simulink library "PTOSim_Lib"  (R2014b)
settings: Solver=ode45  StartTime=0.0  StopTime=10.0  RelTol=1e-3
undefined symbols (not defined in the file): alpha, Amax, Amin, Ap, Beta_e, bf, bg, Cd, D, driveEff, J, k1, k2, omegaBase, omegaInit, pAeq, pAi, pAupper_limit, pBeq, pBi, pBupper_limit, pCprecharge, pDprecharge, pMax, pMin, rho, simu, TgenBase, tot, VC0, VCeq, VD0, VDeq, Vo
libraries: PTOSim_Lib x7, WECSim_Lib x2
settings Model: Creator=sor  LastModifiedBy=sor

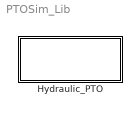
== system PTOSim_Lib ==
  Hydraulic_PTO : Subsystem  RequirementInfo={} %GIDa_f12a42eb_b9cb_4818_b573_b7dee4183a3b

== system PTOSim_Lib/Hydraulic_PTO ==
  Accumulator : Subsystem  Variant=on  mask{pto=0}
      mask prompts: pto "PTO Name"
  Generator : Subsystem  RequirementInfo="{}  %GIDa_30368e1c_dc2a_4605_bb50_ff3a423f2df5"  mask{pto=0}
      mask prompts: pto "PTO Name"
  "Motor " : Subsystem  mask{pto=0}
      mask prompts: pto "PTO Name"
  PTOSIM : Subsystem  RequirementInfo="{}  %GIDa_b8f519ee_1776_4469_9852_74bfa511eadd"  mask{Parameter1=0}
      mask prompts: Parameter1 "pto"
  "Piston " : Subsystem  mask{pto=0}
      mask prompts: pto "PTO Name"
  Piston 1 : PTOSim_Lib/Hydraulic_PTO/Piston    pto=0
  Rectifiying Check Valve : Subsystem  RequirementInfo="{}  %GIDa_a75844df_5079_4f47_95bd_8083cdfec0d7"  mask{pto=0}
      mask prompts: pto "PTO Name"

== system PTOSim_Lib/Hydraulic_PTO/Accumulator ==
  note: 1) Only subsystems can be added as variant choices at this level
      | 2) Blocks cannot be connected at this level as connectivity is
      | automatically determined at simulation, based on the active variant
  Vdot : Inport
  Vdotm : Inport  Port=2
  High Pressure Accumulator : Subsystem  VariantControl=Variant
  Low Pressure Accumulator : Subsystem  VariantControl=Variant1
  Pressure : Outport

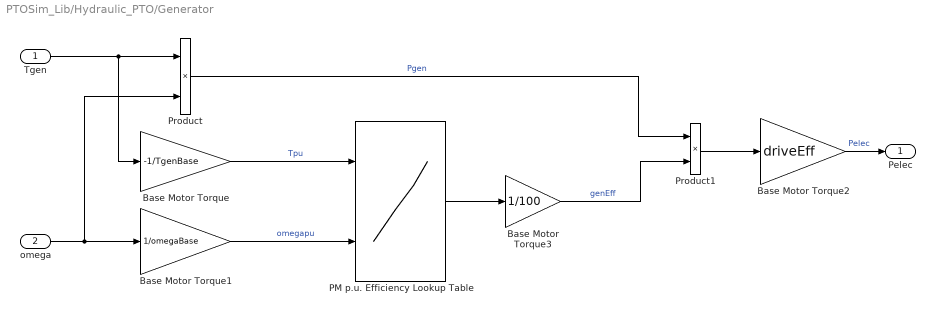
== system PTOSim_Lib/Hydraulic_PTO/Generator ==
  Tgen : Inport
  omega : Inport  Port=2
  Base Motor Torque : Gain  Gain=-1/TgenBase
  Base Motor Torque1 : Gain  Gain=1/omegaBase
  Base Motor Torque2 : Gain  Gain=driveEff
  Base Motor Torque3 : Gain  Gain=1/100
  PM p.u. Efficiency Lookup Table : Lookup_n-D  BreakpointsForDimension1=tot.Tpu(:,1)  BreakpointsForDimension2=tot.omegapu(1,:)  Table=tot.eff  InterpMethod=Flat  InputSameDT=on
  Product : Product  RndMeth=Zero
  Product1 : Product  RndMeth=Zero
  Pelec : Outport
  wires:
  Base Motor Torque2/1 -> Pelec/1  "Pelec"
  Product1/1 -> Base Motor Torque2/1
  Product/1 -> Product1/1  "Pgen"
  Base Motor Torque3/1 -> Product1/2  "genEff"
  PM p.u. Efficiency Lookup Table/1 -> Base Motor Torque3/1
  omega/1 -> Product/2, Base Motor Torque1/1
  Base Motor Torque1/1 -> PM p.u. Efficiency Lookup Table/2  "omegapu"
  Tgen/1 -> Base Motor Torque/1, Product/1
  Base Motor Torque/1 -> PM p.u. Efficiency Lookup Table/1  "Tpu"

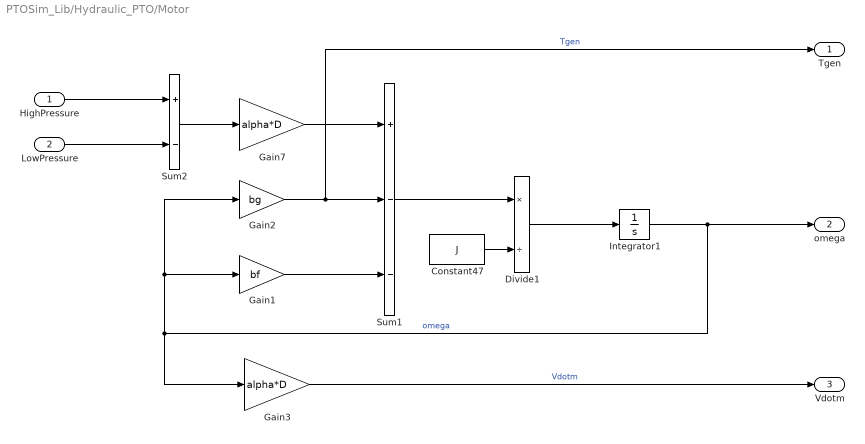
== system PTOSim_Lib/Hydraulic_PTO/Motor  ==
  HighPressure : Inport
  LowPressure : Inport  Port=2
  Constant47 : Constant  Value=J
  Divide1 : Product  Inputs=*/
  Gain1 : Gain  Gain=bf
  Gain2 : Gain  Gain=bg
  Gain3 : Gain  Gain=alpha*D
  Gain7 : Gain  Gain=alpha*D
  Integrator1 : Integrator  InitialCondition=omegaInit
  Sum1 : Sum  Inputs=+--
  Sum2 : Sum  Inputs=+-
  Tgen : Outport
  omega : Outport  Port=2
  Vdotm : Outport  Port=3
  wires:
  Gain7/1 -> Sum1/1
  Gain2/1 -> Tgen/1, Sum1/2  "Tgen"
  Gain1/1 -> Sum1/3
  Sum1/1 -> Divide1/1
  Constant47/1 -> Divide1/2
  Divide1/1 -> Integrator1/1
  Integrator1/1 -> omega/1, Gain3/1, Gain1/1, Gain2/1  "omega"
  Gain3/1 -> Vdotm/1  "Vdotm"
  HighPressure/1 -> Sum2/1
  LowPressure/1 -> Sum2/2
  Sum2/1 -> Gain7/1

== system PTOSim_Lib/Hydraulic_PTO/PTOSIM ==
  zRel : Inport
  zDotRel : Inport  Port=2
  Accumulator : PTOSim_Lib/Hydraulic_PTO/Accumulator  OverrideUsingVariant=Variant  pto=0
  Accumulator1 : PTOSim_Lib/Hydraulic_PTO/Accumulator  OverrideUsingVariant=Variant1  pto=0
  Generator : PTOSim_Lib/Hydraulic_PTO/Generator  pto=0
  "Motor " : PTOSim_Lib/Hydraulic_PTO/Motor   pto=0
  "Piston " : PTOSim_Lib/Hydraulic_PTO/Piston    pto=0
  Rectifiying Check Valve : PTOSim_Lib/Hydraulic_PTO/Rectifiying  Check Valve  pto=0
  Terminator : Terminator
  Fpto : Outport
  wires:
  zRel/1 -> "Piston "/1  "zRel"
  zDotRel/1 -> "Piston "/2  "zDotRel"
  "Piston "/2 -> Rectifiying Check Valve/1  "TopPistonPressure"
  "Piston "/3 -> Rectifiying Check Valve/2  "BottomPistonPressure"
  "Motor "/1 -> Generator/1
  "Motor "/2 -> Generator/2
  "Motor "/3 -> Accumulator/2, Accumulator1/2
  Accumulator/1 -> Rectifiying Check Valve/3, "Motor "/1  "HighPressure"
  Accumulator1/1 -> "Motor "/2, Rectifiying Check Valve/4  "LowPressure"
  Rectifiying Check Valve/1 -> "Piston "/3, Accumulator1/1, Accumulator/1
  Generator/1 -> Terminator/1
  "Piston "/1 -> Fpto/1

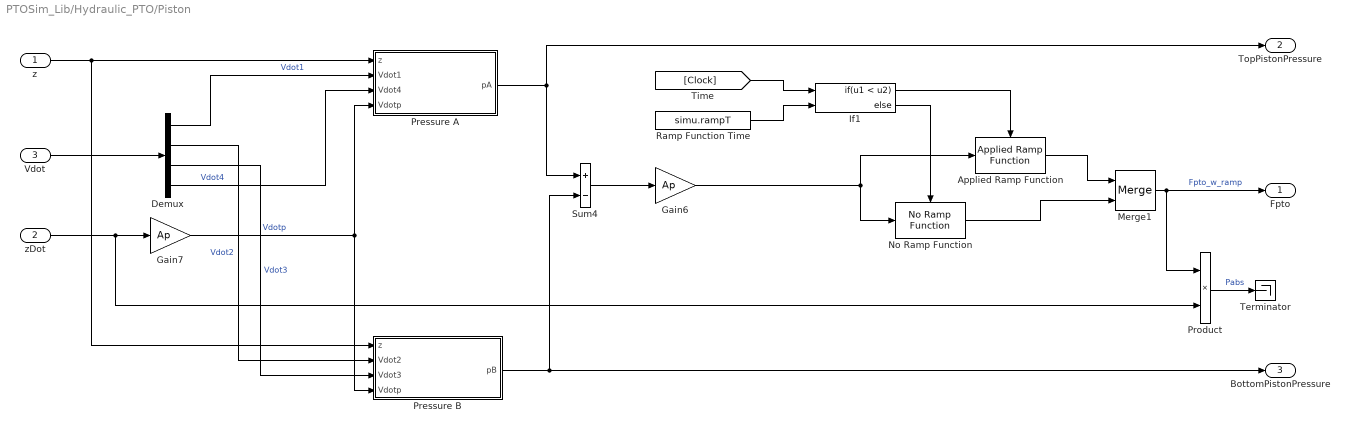
== system PTOSim_Lib/Hydraulic_PTO/Piston  ==
  z : Inport
  zDot : Inport  Port=2
  Vdot : Inport  Port=3
  Applied Ramp Function : WECSim_Lib/Body Elements/Rigid Body/Wave Diffraction and Excitation Force Calculation/Applied Ramp Function
  Demux : Demux
  Gain6 : Gain  Gain=Ap
  Gain7 : Gain  Gain=Ap
  If1 : If  NumInputs=2  IfExpression=u1 < u2
  Merge1 : Merge
  No Ramp Function : WECSim_Lib/Body Elements/Rigid Body/Wave Diffraction and Excitation Force Calculation/No Ramp Function
  Pressure A : Subsystem
  Pressure B : Subsystem  RequirementInfo="{}  %GIDa_18ee15fe_6148_4b69_b054_be19d4b47378"
  Product : Product
  Ramp Function Time : Constant  Value=simu.rampT
  Sum4 : Sum  Inputs=+-
  Terminator : Terminator
  Fpto : Outport
  TopPistonPressure : Outport  Port=2
  BottomPistonPressure : Outport  Port=3
  wires:
  Pressure A/1(pA) -> TopPistonPressure/1, Sum4/1
  Pressure B/1(pB) -> Sum4/2, BottomPistonPressure/1
  Gain7/1 -> Pressure B/4(Vdotp), Pressure A/4(Vdotp)  "Vdotp"
  Gain6/1 -> No Ramp Function/1, Applied Ramp Function/1
  Product/1 -> Terminator/1  "Pabs"
  Vdot/1 -> Demux/1
  z/1 -> Pressure B/1(z), Pressure A/1(z)
  Demux/1 -> Pressure A/2(Vdot1)  "Vdot1"
  Demux/2 -> Pressure B/2(Vdot2)  "Vdot2"
  Demux/3 -> Pressure B/3(Vdot3)  "Vdot3"
  Demux/4 -> Pressure A/3(Vdot4)  "Vdot4"
  Sum4/1 -> Gain6/1
  If1/1 -> Applied Ramp Function/Action
  If1/2 -> No Ramp Function/Action
  Applied Ramp Function/1 -> Merge1/1
  No Ramp Function/1 -> Merge1/2
  Merge1/1 -> Product/1, Fpto/1  "Fpto_w_ramp"
  [Clock] -> If1/1
  Ramp Function Time/1 -> If1/2
  zDot/1 -> Product/2, Gain7/1

== system PTOSim_Lib/Hydraulic_PTO/Rectifiying Check Valve ==
  TopPistonPressure : Inport
  BottomPistonPressure : Inport  Port=2
  HighPressure : Inport  Port=3
  LowPressure : Inport  Port=4
  Bus Creator : BusCreator
  Subsystem : Subsystem  RequirementInfo="{}  %GIDa_43e7490a_26e5_4c96_a755_05599e7ab58d"
  Subsystem1 : Subsystem
  Subsystem2 : Subsystem
  Subsystem3 : Subsystem  RequirementInfo="{}  %GIDa_1d14c02d_1c58_4958_a821_20fe782ea22d"
  Vdot : Outport
  wires:
  TopPistonPressure/1 -> Subsystem3/2(pA), Subsystem/1(pA)
  BottomPistonPressure/1 -> Subsystem2/2(pB), Subsystem1/1(pB)
  HighPressure/1 -> Subsystem1/2(pC), Subsystem/2(pC)
  LowPressure/1 -> Subsystem3/1(pD), Subsystem2/1(pD)
  Subsystem3/1(Vdot4) -> Bus Creator/4  "Vdot4"
  Subsystem2/1(Vdot3) -> Bus Creator/3  "Vdot3"
  Subsystem1/1(Vdot2) -> Bus Creator/2  "Vdot2"
  Subsystem/1(Vdot1) -> Bus Creator/1  "Vdot1"
  Bus Creator/1 -> Vdot/1

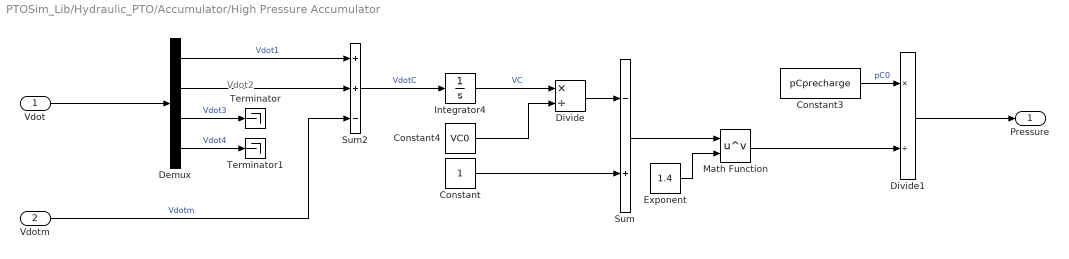
== system PTOSim_Lib/Hydraulic_PTO/Accumulator/High Pressure Accumulator ==
  note: Vdot2
  Vdot : Inport
  Vdotm : Inport  Port=2
  Constant : Constant
  Constant3 : Constant  Value=pCprecharge
  Constant4 : Constant  Value=VC0
  Demux : Demux
  Divide : Product  Inputs=*/
  Divide1 : Product  Inputs=*/
  Exponent : Constant  Value=1.4
  Integrator4 : Integrator  InitialCondition=VCeq
  Math Function : Math  Operator=pow  SaturateOnIntegerOverflow=on
  Sum : Sum  Inputs=-+
  Sum2 : Sum  Inputs=++-
  Terminator : Terminator
  Terminator1 : Terminator
  Pressure : Outport
  wires:
  Sum2/1 -> Integrator4/1  "VdotC"
  Integrator4/1 -> Divide/1  "VC"
  Constant4/1 -> Divide/2
  Constant/1 -> Sum/2
  Divide/1 -> Sum/1
  Exponent/1 -> Math Function/2
  Sum/1 -> Math Function/1
  Math Function/1 -> Divide1/2
  Constant3/1 -> Divide1/1  "pC0"
  Divide1/1 -> Pressure/1
  Vdot/1 -> Demux/1
  Demux/3 -> Terminator/1  "Vdot3"
  Demux/4 -> Terminator1/1  "Vdot4"
  Demux/1 -> Sum2/1  "Vdot1"
  Demux/2 -> Sum2/2
  Vdotm/1 -> Sum2/3  "Vdotm"

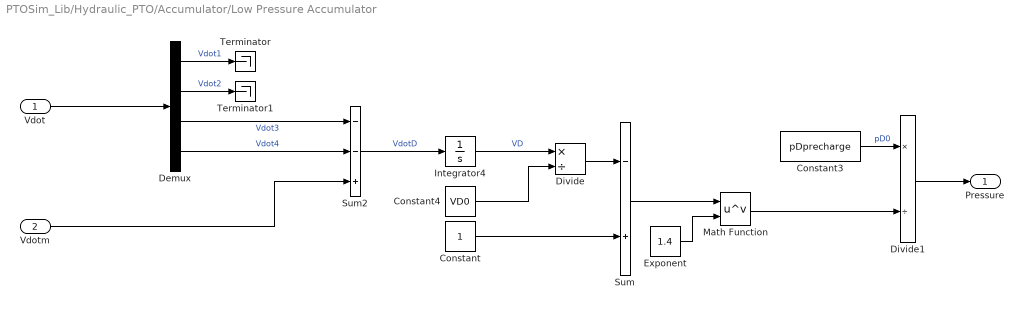
== system PTOSim_Lib/Hydraulic_PTO/Accumulator/Low Pressure Accumulator ==
  Vdot : Inport
  Vdotm : Inport  Port=2
  Constant : Constant
  Constant3 : Constant  Value=pDprecharge
  Constant4 : Constant  Value=VD0
  Demux : Demux
  Divide : Product  Inputs=*/
  Divide1 : Product  Inputs=*/
  Exponent : Constant  Value=1.4
  Integrator4 : Integrator  InitialCondition=VDeq
  Math Function : Math  Operator=pow  SaturateOnIntegerOverflow=on
  Sum : Sum  Inputs=-+
  Sum2 : Sum  Inputs=--+
  Terminator : Terminator
  Terminator1 : Terminator
  Pressure : Outport
  wires:
  Sum2/1 -> Integrator4/1  "VdotD"
  Integrator4/1 -> Divide/1  "VD"
  Constant4/1 -> Divide/2
  Constant/1 -> Sum/2
  Divide/1 -> Sum/1
  Exponent/1 -> Math Function/2
  Sum/1 -> Math Function/1
  Math Function/1 -> Divide1/2
  Constant3/1 -> Divide1/1  "pD0"
  Divide1/1 -> Pressure/1
  Vdot/1 -> Demux/1
  Demux/3 -> Sum2/1  "Vdot3"
  Demux/4 -> Sum2/2  "Vdot4"
  Vdotm/1 -> Sum2/3
  Demux/1 -> Terminator/1  "Vdot1"
  Demux/2 -> Terminator1/1  "Vdot2"

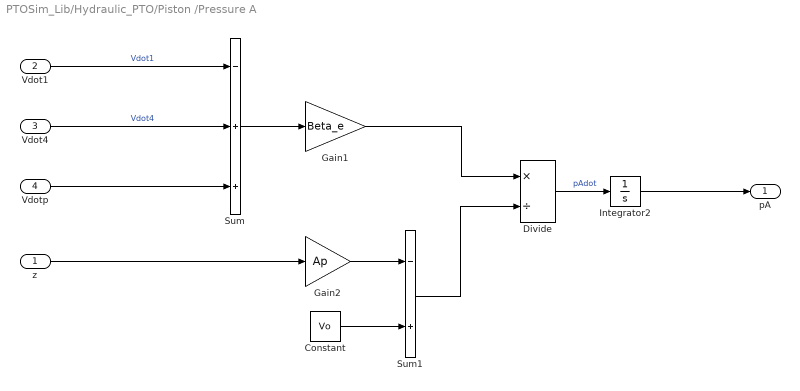
== system PTOSim_Lib/Hydraulic_PTO/Piston /Pressure A ==
  z : Inport
  Vdot1 : Inport  Port=2
  Vdot4 : Inport  Port=3
  Vdotp : Inport  Port=4
  Constant : Constant  Value=Vo
  Divide : Product  Inputs=*/
  Gain1 : Gain  Gain=Beta_e
  Gain2 : Gain  Gain=Ap
  Integrator2 : Integrator  InitialCondition=pAi  UpperSaturationLimit=pAupper_limit  LowerSaturationLimit=pAeq
  Sum : Sum  Inputs=-++
  Sum1 : Sum  Inputs=-+
  pA : Outport
  wires:
  Sum/1 -> Gain1/1
  z/1 -> Gain2/1
  Gain2/1 -> Sum1/1
  Constant/1 -> Sum1/2
  Gain1/1 -> Divide/1
  Sum1/1 -> Divide/2
  Vdot1/1 -> Sum/1  "Vdot1"
  Divide/1 -> Integrator2/1  "pAdot"
  Vdot4/1 -> Sum/2  "Vdot4"
  Integrator2/1 -> pA/1
  Vdotp/1 -> Sum/3

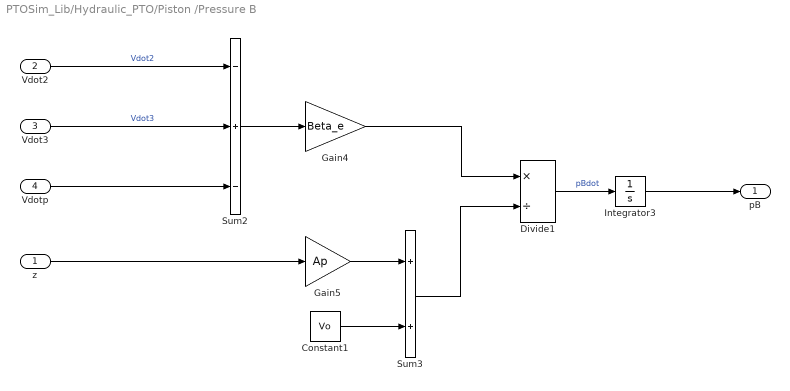
== system PTOSim_Lib/Hydraulic_PTO/Piston /Pressure B ==
  z : Inport
  Vdot2 : Inport  Port=2
  Vdot3 : Inport  Port=3
  Vdotp : Inport  Port=4
  Constant1 : Constant  Value=Vo
  Divide1 : Product  Inputs=*/
  Gain4 : Gain  Gain=Beta_e
  Gain5 : Gain  Gain=Ap
  Integrator3 : Integrator  InitialCondition=pBi  UpperSaturationLimit=pBupper_limit  LowerSaturationLimit=pBeq
  Sum2 : Sum  Inputs=-+-
  Sum3 : Sum
  pB : Outport
  wires:
  Sum2/1 -> Gain4/1
  z/1 -> Gain5/1
  Gain5/1 -> Sum3/1
  Constant1/1 -> Sum3/2
  Gain4/1 -> Divide1/1
  Sum3/1 -> Divide1/2
  Divide1/1 -> Integrator3/1  "pBdot"
  Vdot2/1 -> Sum2/1  "Vdot2"
  Vdot3/1 -> Sum2/2  "Vdot3"
  Integrator3/1 -> pB/1
  Vdotp/1 -> Sum2/3

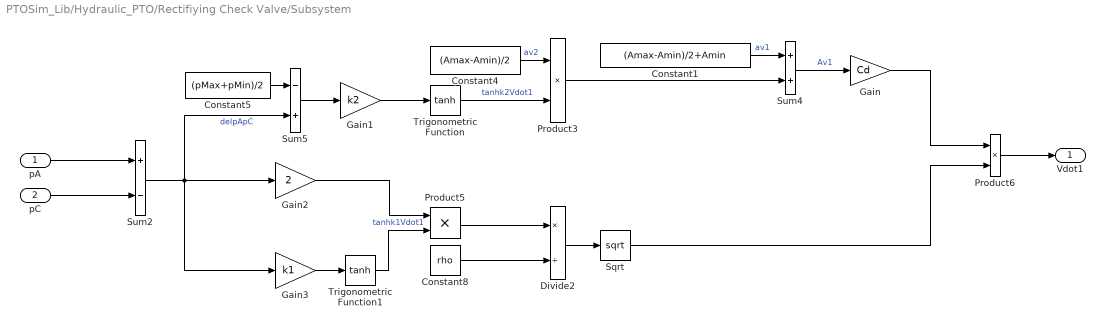
== system PTOSim_Lib/Hydraulic_PTO/Rectifiying Check Valve/Subsystem ==
  pA : Inport
  pC : Inport  Port=2
  Constant1 : Constant  Value=(Amax-Amin)/2+Amin
  Constant4 : Constant  Value=(Amax-Amin)/2
  Constant5 : Constant  Value=(pMax+pMin)/2
  Constant8 : Constant  Value=rho
  Divide2 : Product  Inputs=*/
  Gain : Gain  Gain=Cd
  Gain1 : Gain  Gain=k2
  Gain2 : Gain  Gain=2
  Gain3 : Gain  Gain=k1
  Product3 : Product
  Product5 : Product
  Product6 : Product
  Sqrt : Sqrt  SaturateOnIntegerOverflow=on
  Sum2 : Sum  Inputs=+-
  Sum4 : Sum
  Sum5 : Sum  Inputs=-+
  Trigonometric Function : Trigonometry  Operator=tanh
  Trigonometric Function1 : Trigonometry  Operator=tanh
  Vdot1 : Outport
  wires:
  Gain1/1 -> Trigonometric Function/1
  Trigonometric Function/1 -> Product3/2  "tanhk2Vdot1"
  Product3/1 -> Sum4/2
  Sum5/1 -> Gain1/1
  Sum4/1 -> Gain/1  "Av1"
  Gain3/1 -> Trigonometric Function1/1
  Gain2/1 -> Product5/1
  Trigonometric Function1/1 -> Product5/2  "tanhk1Vdot1"
  Sqrt/1 -> Product6/2
  Gain/1 -> Product6/1
  Constant8/1 -> Divide2/2
  Product5/1 -> Divide2/1
  Divide2/1 -> Sqrt/1
  pA/1 -> Sum2/1
  pC/1 -> Sum2/2
  Product6/1 -> Vdot1/1
  Constant4/1 -> Product3/1  "av2"
  Constant5/1 -> Sum5/1
  Constant1/1 -> Sum4/1  "av1"
  Sum2/1 -> Gain3/1, Sum5/2, Gain2/1  "delpApC"

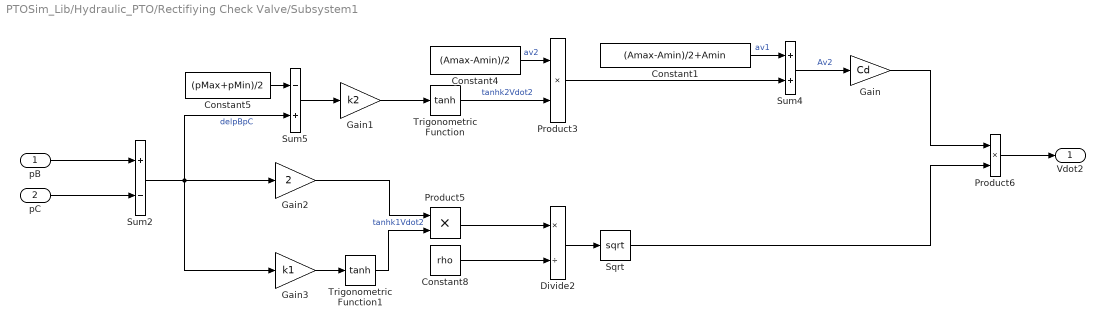
== system PTOSim_Lib/Hydraulic_PTO/Rectifiying Check Valve/Subsystem1 ==
  pB : Inport
  pC : Inport  Port=2
  Constant1 : Constant  Value=(Amax-Amin)/2+Amin
  Constant4 : Constant  Value=(Amax-Amin)/2
  Constant5 : Constant  Value=(pMax+pMin)/2
  Constant8 : Constant  Value=rho
  Divide2 : Product  Inputs=*/
  Gain : Gain  Gain=Cd
  Gain1 : Gain  Gain=k2
  Gain2 : Gain  Gain=2
  Gain3 : Gain  Gain=k1
  Product3 : Product
  Product5 : Product
  Product6 : Product
  Sqrt : Sqrt  SaturateOnIntegerOverflow=on
  Sum2 : Sum  Inputs=+-
  Sum4 : Sum
  Sum5 : Sum  Inputs=-+
  Trigonometric Function : Trigonometry  Operator=tanh
  Trigonometric Function1 : Trigonometry  Operator=tanh
  Vdot2 : Outport
  wires:
  Gain1/1 -> Trigonometric Function/1
  Trigonometric Function/1 -> Product3/2  "tanhk2Vdot2"
  Product3/1 -> Sum4/2
  Sum5/1 -> Gain1/1
  Sum4/1 -> Gain/1  "Av2"
  Gain3/1 -> Trigonometric Function1/1
  Gain2/1 -> Product5/1
  Trigonometric Function1/1 -> Product5/2  "tanhk1Vdot2"
  Sqrt/1 -> Product6/2
  Gain/1 -> Product6/1
  Constant8/1 -> Divide2/2
  Product5/1 -> Divide2/1
  Divide2/1 -> Sqrt/1
  pB/1 -> Sum2/1
  pC/1 -> Sum2/2
  Product6/1 -> Vdot2/1
  Constant4/1 -> Product3/1  "av2"
  Constant5/1 -> Sum5/1
  Constant1/1 -> Sum4/1  "av1"
  Sum2/1 -> Gain3/1, Sum5/2, Gain2/1  "delpBpC"

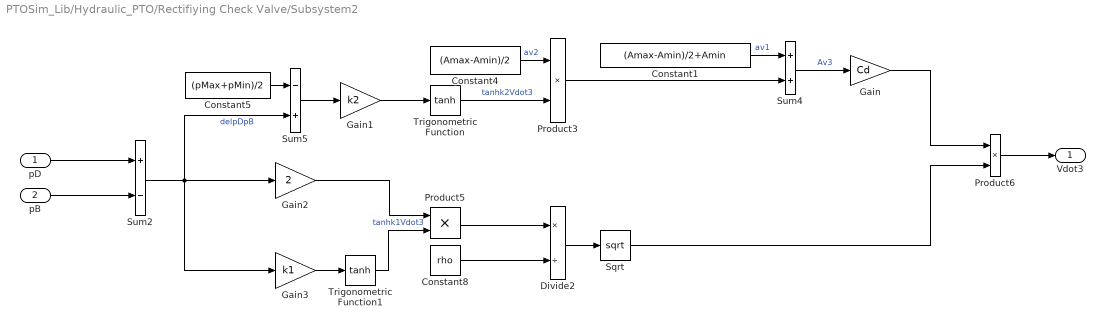
== system PTOSim_Lib/Hydraulic_PTO/Rectifiying Check Valve/Subsystem2 ==
  pD : Inport
  pB : Inport  Port=2
  Constant1 : Constant  Value=(Amax-Amin)/2+Amin
  Constant4 : Constant  Value=(Amax-Amin)/2
  Constant5 : Constant  Value=(pMax+pMin)/2
  Constant8 : Constant  Value=rho
  Divide2 : Product  Inputs=*/
  Gain : Gain  Gain=Cd
  Gain1 : Gain  Gain=k2
  Gain2 : Gain  Gain=2
  Gain3 : Gain  Gain=k1
  Product3 : Product
  Product5 : Product
  Product6 : Product
  Sqrt : Sqrt  SaturateOnIntegerOverflow=on
  Sum2 : Sum  Inputs=+-
  Sum4 : Sum
  Sum5 : Sum  Inputs=-+
  Trigonometric Function : Trigonometry  Operator=tanh
  Trigonometric Function1 : Trigonometry  Operator=tanh
  Vdot3 : Outport
  wires:
  Gain1/1 -> Trigonometric Function/1
  Trigonometric Function/1 -> Product3/2  "tanhk2Vdot3"
  Product3/1 -> Sum4/2
  Sum5/1 -> Gain1/1
  Sum4/1 -> Gain/1  "Av3"
  Gain3/1 -> Trigonometric Function1/1
  Gain2/1 -> Product5/1
  Trigonometric Function1/1 -> Product5/2  "tanhk1Vdot3"
  Sqrt/1 -> Product6/2
  Gain/1 -> Product6/1
  Constant8/1 -> Divide2/2
  Product5/1 -> Divide2/1
  Divide2/1 -> Sqrt/1
  pD/1 -> Sum2/1
  pB/1 -> Sum2/2
  Product6/1 -> Vdot3/1
  Constant4/1 -> Product3/1  "av2"
  Constant5/1 -> Sum5/1
  Constant1/1 -> Sum4/1  "av1"
  Sum2/1 -> Gain3/1, Sum5/2, Gain2/1  "delpDpB"

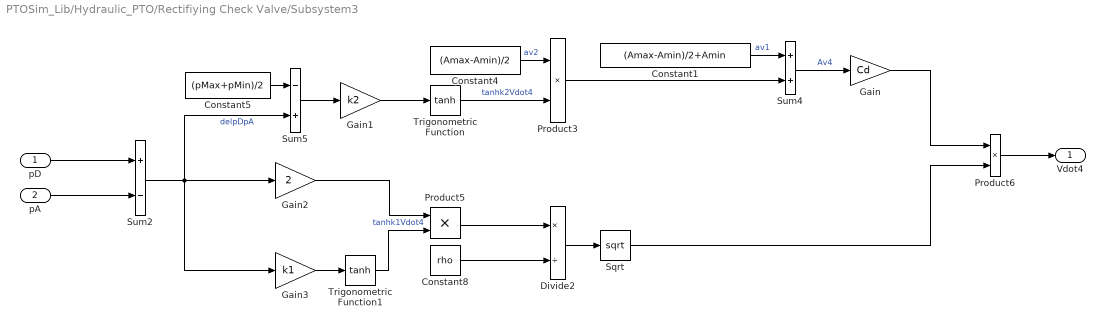
== system PTOSim_Lib/Hydraulic_PTO/Rectifiying Check Valve/Subsystem3 ==
  pD : Inport
  pA : Inport  Port=2
  Constant1 : Constant  Value=(Amax-Amin)/2+Amin
  Constant4 : Constant  Value=(Amax-Amin)/2
  Constant5 : Constant  Value=(pMax+pMin)/2
  Constant8 : Constant  Value=rho
  Divide2 : Product  Inputs=*/
  Gain : Gain  Gain=Cd
  Gain1 : Gain  Gain=k2
  Gain2 : Gain  Gain=2
  Gain3 : Gain  Gain=k1
  Product3 : Product
  Product5 : Product
  Product6 : Product
  Sqrt : Sqrt  SaturateOnIntegerOverflow=on
  Sum2 : Sum  Inputs=+-
  Sum4 : Sum
  Sum5 : Sum  Inputs=-+
  Trigonometric Function : Trigonometry  Operator=tanh
  Trigonometric Function1 : Trigonometry  Operator=tanh
  Vdot4 : Outport
  wires:
  Gain1/1 -> Trigonometric Function/1
  Trigonometric Function/1 -> Product3/2  "tanhk2Vdot4"
  Product3/1 -> Sum4/2
  Sum5/1 -> Gain1/1
  Sum4/1 -> Gain/1  "Av4"
  Gain3/1 -> Trigonometric Function1/1
  Gain2/1 -> Product5/1
  Trigonometric Function1/1 -> Product5/2  "tanhk1Vdot4"
  Sqrt/1 -> Product6/2
  Gain/1 -> Product6/1
  Constant8/1 -> Divide2/2
  Product5/1 -> Divide2/1
  Divide2/1 -> Sqrt/1
  pD/1 -> Sum2/1
  pA/1 -> Sum2/2
  Product6/1 -> Vdot4/1
  Constant4/1 -> Product3/1  "av2"
  Constant5/1 -> Sum5/1
  Constant1/1 -> Sum4/1  "av1"
  Sum2/1 -> Gain3/1, Sum5/2, Gain2/1  "delpDpA"
